simulink model "estimator_ukf"  (Simulink 7.0)
settings: Solver=FixedStepDiscrete  StartTime=1  StopTime=10.0  FixedStep=ts  RelTol=1e-3
undefined symbols (not defined in the file): c, m, magnitude, n, P0, Q, R, ROBOT, ts, W, WM, X0
libraries: simulink x5, robotics x5
settings Model: Creator=raje_ra  LastModifiedBy=raje_ra

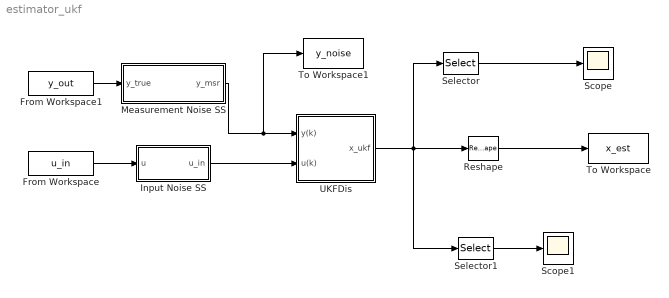
== system estimator_ukf ==
  From Workspace : FromWorkspace  VariableName=u_in  SampleTime=0
  From Workspace1 : FromWorkspace  VariableName=y_out  SampleTime=0
  Input Noise SS : Subsystem
  Measurement Noise SS : Subsystem
  Reshape : Reshape
  Scope : Scope
      settings: YMin=-2e-009  YMax=1.25e-009
  Scope1 : Scope
      settings: TimeRange=10
  Selector : Selector  InputPortWidth=62  IndexOptions=Index vector (dialog)  Indices=[1:6]  OutputSizes=1
  Selector1 : Selector  InputPortWidth=62  IndexOptions=Index vector (dialog)  Indices=[32:37]  OutputSizes=1
  To Workspace : ToWorkspace  VariableName=x_est  SampleTime=-1  SaveFormat=Structure With Time
  To Workspace1 : ToWorkspace  VariableName=y_noise  SampleTime=-1  SaveFormat=Structure With Time
  UKFDis : Subsystem
  wires:
  UKFDis/1(x_ukf) -> Selector/1, Selector1/1, Reshape/1
  From Workspace1/1 -> Measurement Noise SS/1(y_true)
  From Workspace/1 -> Input Noise SS/1(u)
  Selector/1 -> Scope/1
  Selector1/1 -> Scope1/1
  Reshape/1 -> To Workspace/1
  Measurement Noise SS/1(y_msr) -> UKFDis/1(y(k)), To Workspace1/1
  Input Noise SS/1(u_in) -> UKFDis/2(u(k))

== system estimator_ukf/Input Noise SS ==
  note: Noise with Sandard Deviation 1e-1 is added to inputs
  u : Inport  OutDataType=sfix(16)  OutScaling=2^0
  Band-Limited White Noise1 : simulink/Sources/Band-Limited White Noise  SystemSampleTime=-1  Cov=[1e-5]  Ts=ts  seed=[23341]
  Sum : Sum  Inputs=|++  OutDataType=sfix(16)  OutScaling=2^0
  u_in : Outport
  wires:
  Band-Limited White Noise1/1 -> Sum/2
  Sum/1 -> u_in/1
  u/1 -> Sum/1

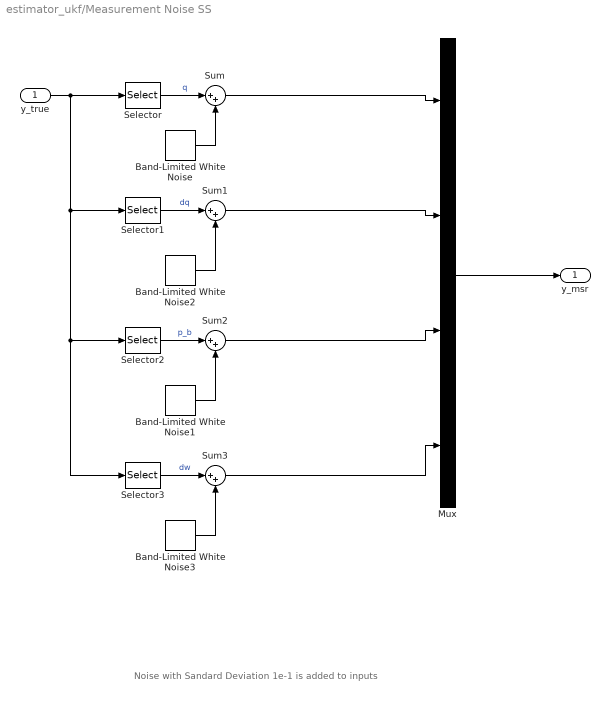
== system estimator_ukf/Measurement Noise SS ==
  note: Noise with Sandard Deviation 1e-1 is added to inputs
  y_true : Inport  OutDataType=sfix(16)  OutScaling=2^0
  Band-Limited White Noise : simulink/Sources/Band-Limited White Noise  SystemSampleTime=-1  Cov=[1e-9]  Ts=ts  seed=[23341]
  Band-Limited White Noise1 : simulink/Sources/Band-Limited White Noise  SystemSampleTime=-1  Cov=[1e-5]  Ts=ts  seed=[23341]
  Band-Limited White Noise2 : simulink/Sources/Band-Limited White Noise  SystemSampleTime=-1  Cov=[1e-7]  Ts=ts  seed=[23341]
  Band-Limited White Noise3 : simulink/Sources/Band-Limited White Noise  SystemSampleTime=-1  Cov=[1e-7]  Ts=ts  seed=[23341]
  Mux : Mux
  Selector : Selector  InputPortWidth=m  IndexOptions=Index vector (dialog)  Indices=[1:25]  OutputSizes=1
  Selector1 : Selector  InputPortWidth=m  IndexOptions=Index vector (dialog)  Indices=[26:50]  OutputSizes=1
  Selector2 : Selector  InputPortWidth=m  IndexOptions=Index vector (dialog)  Indices=[51:53]  OutputSizes=1
  Selector3 : Selector  InputPortWidth=m  IndexOptions=Index vector (dialog)  Indices=[54:56]  OutputSizes=1
  Sum{,1..3} (4 alike) : Sum  Inputs=|++  OutDataType=sfix(16)  OutScaling=2^0
  y_msr : Outport
  wires:
  Mux/1 -> y_msr/1
  Sum3/1 -> Mux/4
  Sum2/1 -> Mux/3
  Sum1/1 -> Mux/2
  Sum/1 -> Mux/1
  Selector3/1 -> Sum3/1  "dw"
  Band-Limited White Noise3/1 -> Sum3/2
  Selector2/1 -> Sum2/1  "p_b"
  Band-Limited White Noise1/1 -> Sum2/2
  Band-Limited White Noise2/1 -> Sum1/2
  Selector1/1 -> Sum1/1  "dq"
  Selector/1 -> Sum/1  "q"
  y_true/1 -> Selector3/1, Selector2/1, Selector1/1, Selector/1
  Band-Limited White Noise/1 -> Sum/2

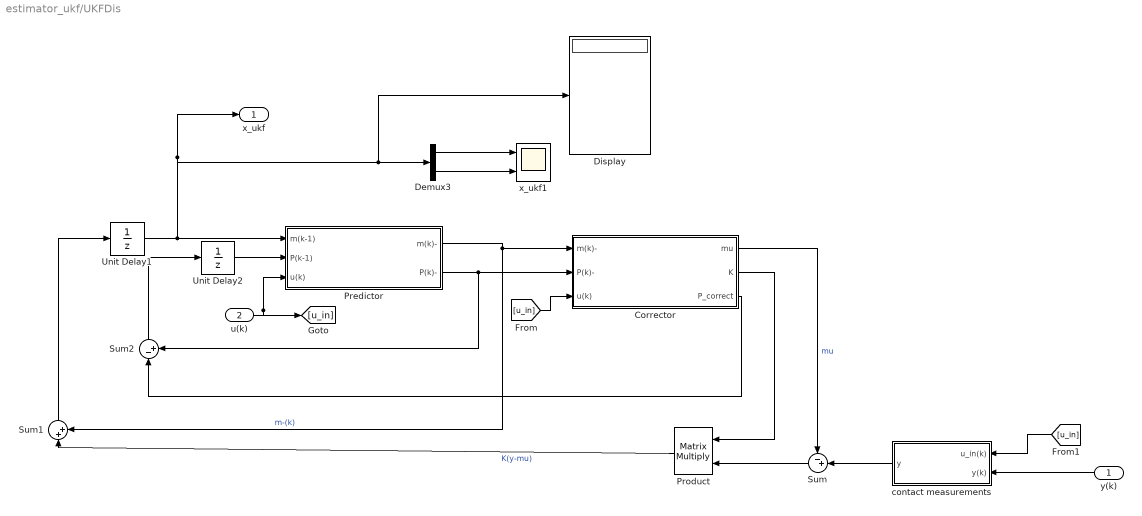
== system estimator_ukf/UKFDis ==
  y(k) : Inport  Orientation=left
  u(k) : Inport  Port=2
  Corrector : Subsystem
  Demux3 : Demux  Outputs=2
  Display : Display
  Predictor : Subsystem
  Product : Product  Orientation=left  Multiplication=Matrix(*)  OutDataType=sfix(16)  OutScaling=2^0  RndMeth=Zero
  Sum : Sum  Orientation=left  Inputs=-+|  OutDataType=sfix(16)  OutScaling=2^0
  Sum1 : Sum  Orientation=up  Inputs=|++  OutDataType=sfix(16)  OutScaling=2^0
  Sum2 : Sum  Orientation=up  Inputs=|-+  OutDataType=sfix(16)  OutScaling=2^0
  Unit Delay1 : UnitDelay  X0=X0  SampleTime=-1
  Unit Delay2 : UnitDelay  X0=P0  SampleTime=-1
  contact measurements : Subsystem  Orientation=left
  x_ukf1 : Scope  NumInputPorts=2
      settings: TimeRange=0.1  YMin=-22.5~-1.25  YMax=12.5~1.5  SaveName=ScopeData2
  x_ukf : Outport  OutDataType=sfix(16)  OutScaling=2^0
  wires:
  Demux3/1 -> x_ukf1/1
  Demux3/2 -> x_ukf1/2
  Sum1/1 -> Unit Delay1/1
  Unit Delay1/1 -> x_ukf/1, Demux3/1, Display/1, Predictor/1(m(k-1))
  Predictor/1(m(k)-) -> Sum1/2, Corrector/1(m(k)-)  "m-(k)"
  Predictor/2(P(k)-) -> Corrector/2(P(k)-), Sum2/2
  Corrector/1(mu) -> Sum/1  "mu"
  Corrector/2(K) -> Product/1
  Sum/1 -> Product/2
  Product/1 -> Sum1/1  "K(y-mu)"
  Unit Delay2/1 -> Predictor/2(P(k-1))
  Corrector/3(P_correct) -> Sum2/1
  Sum2/1 -> Unit Delay2/1
  u(k)/1 -> Predictor/3(u(k)), [u_in]
  [u_in] -> Corrector/3(u(k))
  contact measurements/1(y) -> Sum/2
  [u_in] -> contact measurements/1(u_in(k))
  y(k)/1 -> contact measurements/2(y(k))

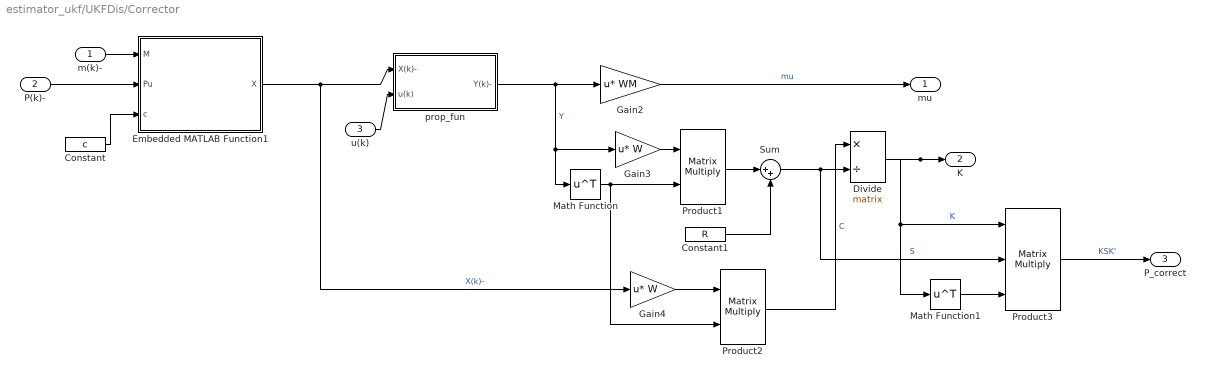
== system estimator_ukf/UKFDis/Corrector ==
  m(k)- : Inport
  P(k)- : Inport  Port=2
  u(k) : Inport  Port=3
  Constant : Constant  Value=c  OutDataType=sfix(16)  OutScaling=2^0
  Constant1 : Constant  Value=R  OutDataType=sfix(16)  OutScaling=2^0
  Divide : Product  Inputs=*/  Multiplication=Matrix(*)  OutDataType=sfix(16)  OutScaling=2^-10
  Embedded MATLAB Function1 : Stateflow chart
  Gain2 : Gain  Gain=WM  Multiplication=Matrix(u*K)  ParameterDataType=sfix(16)  ParameterScaling=2^0  OutDataType=sfix(16)  OutScaling=2^0
  Gain3 : Gain  Gain=W  Multiplication=Matrix(u*K)  ParameterDataType=sfix(16)  ParameterScaling=2^0  OutDataType=sfix(16)  OutScaling=2^0
  Gain4 : Gain  Gain=W  Multiplication=Matrix(u*K)  ParameterDataType=sfix(16)  ParameterScaling=2^0  OutDataType=sfix(16)  OutScaling=2^0
  Math Function : Math  Operator=transpose  OutDataType=sfix(16)  OutScaling=2^0  SaturateOnIntegerOverflow=on
  Math Function1 : Math  Operator=transpose  OutDataType=sfix(16)  OutScaling=2^0  SaturateOnIntegerOverflow=on
  Product1 : Product  Multiplication=Matrix(*)  OutDataType=sfix(16)  OutScaling=2^0  RndMeth=Zero
  Product2 : Product  Multiplication=Matrix(*)  OutDataType=sfix(16)  OutScaling=2^0  RndMeth=Zero
  Product3 : Product  Inputs=3  Multiplication=Matrix(*)  OutDataType=sfix(16)  OutScaling=2^0  RndMeth=Zero
  Sum : Sum  Inputs=|++  OutDataType=sfix(16)  OutScaling=2^0
  prop_fun : Subsystem
  mu : Outport
  K : Outport  Port=2
  P_correct : Outport  Port=3
  wires:
  u(k)/1 -> prop_fun/2(u(k))
  m(k)-/1 -> Embedded MATLAB Function1/1(M)
  P(k)-/1 -> Embedded MATLAB Function1/2(Pu)
  Constant/1 -> Embedded MATLAB Function1/3(c)
  Embedded MATLAB Function1/1(X) -> prop_fun/1(X(k)-), Gain4/1  "X(k)-"
  prop_fun/1(Y(k)-) -> Gain2/1, Gain3/1, Math Function/1  "Y"
  Gain2/1 -> mu/1  "mu"
  Gain3/1 -> Product1/1
  Math Function/1 -> Product1/2, Product2/2
  Product1/1 -> Sum/1
  Constant1/1 -> Sum/2
  Gain4/1 -> Product2/1
  Product2/1 -> Divide/1  "C"
  Sum/1 -> Divide/2, Product3/2  "S"
  Divide/1 -> K/1, Product3/1, Math Function1/1  "K"
  Math Function1/1 -> Product3/3
  Product3/1 -> P_correct/1  "KSK'"

== system estimator_ukf/UKFDis/Predictor ==
  m(k-1) : Inport
  P(k-1) : Inport  Port=2
  u(k) : Inport  Port=3
  Constant : Constant  Value=c  OutDataType=sfix(16)  OutScaling=2^0
  Constant1 : Constant  Value=Q  OutDataType=sfix(16)  OutScaling=2^0
  Embedded MATLAB Function1 : Stateflow chart
  Gain1 : Gain  Gain=WM  Multiplication=Matrix(u*K)  ParameterDataType=sfix(16)  ParameterScaling=2^0  OutDataType=sfix(16)  OutScaling=2^0
  Gain2 : Gain  Gain=W  Multiplication=Matrix(u*K)  ParameterDataType=sfix(16)  ParameterScaling=2^0  OutDataType=sfix(16)  OutScaling=2^0
  Math Function : Math  Operator=transpose  OutDataType=sfix(16)  OutScaling=2^0  SaturateOnIntegerOverflow=on
  Product2 : Product  Multiplication=Matrix(*)  OutDataType=sfix(16)  OutScaling=2^0  RndMeth=Zero
  Sum : Sum  Inputs=|++  OutDataType=sfix(16)  OutScaling=2^0
  prop_fun : Subsystem
  m(k)- : Outport
  P(k)- : Outport  Port=2
  wires:
  u(k)/1 -> prop_fun/2(u(k))
  Embedded MATLAB Function1/1(X) -> prop_fun/1(X(k-1))  "X(k-1)"
  Gain2/1 -> Product2/1
  Math Function/1 -> Product2/2
  Product2/1 -> Sum/1
  Constant1/1 -> Sum/2
  Sum/1 -> P(k)-/1
  Constant/1 -> Embedded MATLAB Function1/3(c)
  m(k-1)/1 -> Embedded MATLAB Function1/1(M)
  P(k-1)/1 -> Embedded MATLAB Function1/2(Pu)
  Gain1/1 -> m(k)-/1
  prop_fun/1(X(k)_hat) -> Gain2/1, Math Function/1, Gain1/1  "X(k)_hat"

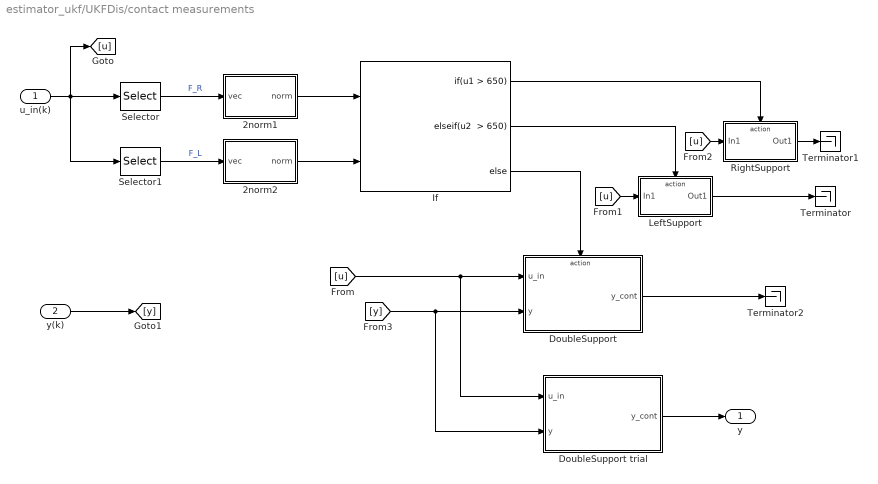
== system estimator_ukf/UKFDis/contact measurements ==
  u_in(k) : Inport
  y(k) : Inport  Port=2
  2norm1 : Subsystem
  2norm2 : Subsystem
  DoubleSupport : Subsystem  TreatAsAtomicUnit=on
  DoubleSupport trial : Subsystem  TreatAsAtomicUnit=on
  If : If  NumInputs=2  IfExpression=u1 > 650  ElseIfExpressions="u2  > 650"
  LeftSupport : Subsystem  TreatAsAtomicUnit=on
  RightSupport : Subsystem  TreatAsAtomicUnit=on
  Selector : Selector  InputPortWidth=37  IndexOptions=Index vector (dialog)  Indices=[1:3]  OutputSizes=1
  Selector1 : Selector  InputPortWidth=37  IndexOptions=Index vector (dialog)  Indices=[4:6]  OutputSizes=1
  Terminator : Terminator
  Terminator1 : Terminator
  Terminator2 : Terminator
  y : Outport
  wires:
  [y] -> DoubleSupport/2(y), DoubleSupport trial/2(y)
  y(k)/1 -> [y]
  [u] -> RightSupport/1(In1)
  [u] -> LeftSupport/1(In1)
  If/2 -> LeftSupport/Action
  If/3 -> DoubleSupport/Action
  u_in(k)/1 -> [u], Selector1/1, Selector/1
  If/1 -> RightSupport/Action
  2norm2/1(norm) -> If/2
  2norm1/1(norm) -> If/1
  Selector1/1 -> 2norm2/1(vec)  "F_L"
  Selector/1 -> 2norm1/1(vec)  "F_R"
  [u] -> DoubleSupport/1(u_in), DoubleSupport trial/1(u_in)
  RightSupport/1(Out1) -> Terminator1/1
  LeftSupport/1(Out1) -> Terminator/1
  DoubleSupport/1(y_cont) -> Terminator2/1
  DoubleSupport trial/1(y_cont) -> y/1

== system estimator_ukf/UKFDis/Corrector/prop_fun ==
  X(k)- : Inport
  u(k) : Inport  Port=2
  F(X) : Subsystem  TreatAsAtomicUnit=on
  Y(k)- : Outport
  wires:
  u(k)/1 -> F(X)/2(u(k))
  X(k)-/1 -> F(X)/1(X(k)-)
  F(X)/1(Y(k)-) -> Y(k)-/1

== system estimator_ukf/UKFDis/Predictor/prop_fun ==
  note: 1)Forward Euler Integration: x(k) = x(k-1) s*f(x(k-1))
  X(k-1) : Inport
  u(k) : Inport  Port=2
  F(X) : Subsystem  TreatAsAtomicUnit=on
  Gain3 : Gain  Gain=ts  ParameterDataType=sfix(16)  ParameterScaling=2^0  OutDataType=sfix(16)  OutScaling=2^0
  Sum1 : Sum  Inputs=|++  OutDataType=sfix(16)  OutScaling=2^0
  X(k)_hat : Outport
  wires:
  u(k)/1 -> F(X)/2(u(k))
  Sum1/1 -> X(k)_hat/1
  X(k-1)/1 -> Sum1/2, F(X)/1(X(k-1))
  F(X)/1(F(X)) -> Gain3/1
  Gain3/1 -> Sum1/1

== system estimator_ukf/UKFDis/contact measurements/2norm1 ==
  vec : Inport
  Math Function : Math  Operator=magnitude^2  OutDataType=sfix(16)  OutScaling=2^0  SaturateOnIntegerOverflow=on
  Math Function1 : Math  Operator=sqrt  OutDataType=sfix(16)  OutScaling=2^0  SaturateOnIntegerOverflow=on
  Sum of Elements : Sum  Inputs=+  OutDataType=sfix(16)  OutScaling=2^-10
  norm : Outport
  wires:
  Math Function/1 -> Sum of Elements/1
  Sum of Elements/1 -> Math Function1/1
  vec/1 -> Math Function/1
  Math Function1/1 -> norm/1

== system estimator_ukf/UKFDis/contact measurements/2norm2 ==
  vec : Inport
  Math Function : Math  Operator=magnitude^2  OutDataType=sfix(16)  OutScaling=2^0  SaturateOnIntegerOverflow=on
  Math Function1 : Math  Operator=sqrt  OutDataType=sfix(16)  OutScaling=2^0  SaturateOnIntegerOverflow=on
  Sum of Elements : Sum  Inputs=+  OutDataType=sfix(16)  OutScaling=2^-10
  norm : Outport
  wires:
  Math Function1/1 -> norm/1
  vec/1 -> Math Function/1
  Sum of Elements/1 -> Math Function1/1
  Math Function/1 -> Sum of Elements/1

== system estimator_ukf/UKFDis/contact measurements/DoubleSupport ==
  u_in : Inport  OutDataType=sfix(16)  OutScaling=2^0
  y : Inport  Port=2  OutDataType=sfix(16)  OutScaling=2^0
  Action Port : ActionPort  ActionType=else
  Constant : Constant  Value=zeros(12,1)  VectorParams1D=off  OutDataType=sfix(16)  OutScaling=2^0
  Matrix Concatenate : Concatenate  Mode=Multidimensional array
  Terminator : Terminator
  y_cont : Outport  OutDataType=sfix(16)  OutScaling=2^0
  wires:
  y/1 -> Matrix Concatenate/1
  Constant/1 -> Matrix Concatenate/2
  Matrix Concatenate/1 -> y_cont/1
  u_in/1 -> Terminator/1

== system estimator_ukf/UKFDis/contact measurements/DoubleSupport trial ==
  u_in : Inport  OutDataType=sfix(16)  OutScaling=2^0
  y : Inport  Port=2  OutDataType=sfix(16)  OutScaling=2^0
  Constant velocities : Constant  Value=zeros(12,1)  VectorParams1D=off  OutDataType=sfix(16)  OutScaling=2^0
  Constant z foot : Constant  Value=zeros(2,1)  VectorParams1D=off  OutDataType=sfix(16)  OutScaling=2^0
  Matrix Concatenate : Concatenate  NumInputs=3  Mode=Multidimensional array
  Selector : Selector  InputPortWidth=70  IndexOptions=Index vector (dialog)  Indices=[1:68]  OutputSizes=1
  Terminator : Terminator
  y_cont : Outport  OutDataType=sfix(16)  OutScaling=2^0
  wires:
  u_in/1 -> Terminator/1
  Matrix Concatenate/1 -> Selector/1
  Constant velocities/1 -> Matrix Concatenate/2
  y/1 -> Matrix Concatenate/1
  Constant z foot/1 -> Matrix Concatenate/3
  Selector/1 -> y_cont/1

== system estimator_ukf/UKFDis/contact measurements/LeftSupport ==
  In1 : Inport  OutDataType=sfix(16)  OutScaling=2^0
  Action Port : ActionPort  ActionType=elseif
  Out1 : Outport  OutDataType=sfix(16)  OutScaling=2^0
  wires:
  In1/1 -> Out1/1

== system estimator_ukf/UKFDis/contact measurements/RightSupport ==
  In1 : Inport  OutDataType=sfix(16)  OutScaling=2^0
  Action Port : ActionPort  ActionType=then
  Out1 : Outport  OutDataType=sfix(16)  OutScaling=2^0
  wires:
  In1/1 -> Out1/1

== system estimator_ukf/UKFDis/Corrector/prop_fun/F(X) ==
  X(k)- : Inport  OutDataType=sfix(16)  OutScaling=2^0
  u(k) : Inport  Port=2  OutDataType=sfix(16)  OutScaling=2^0
  Assignment : Assignment  NumberOfDimensions=2  IndexOptions=Assign all,Index vector (port)  Indices=1,1  OutputSizes=2,2
  Constant : Constant  Value=zeros(m+12,2*n+1)  VectorParams1D=off  OutDataType=sfix(16)  OutScaling=2^0  SampleTime=-1
  Display : Display
  For Iterator : ForIterator  ResetStates=reset  IterationLimit=2*n +1  IterationVariableDataType=double
  Measurements : Subsystem
  Selector : Selector  NumberOfDimensions=2  IndexOptions=Select all,Index vector (port)  Indices=[1 3],1  OutputSizes=1,1
  Y(k)- : Outport  OutDataType=sfix(16)  OutScaling=2^0
  wires:
  u(k)/1 -> Measurements/2(u)
  Constant/1 -> Assignment/1
  Assignment/1 -> Y(k)-/1
  Measurements/1(y) -> Assignment/2
  Selector/1 -> Measurements/1(x)
  For Iterator/1 -> Display/1, Assignment/3, Selector/2
  X(k)-/1 -> Selector/1

== system estimator_ukf/UKFDis/Predictor/prop_fun/F(X) ==
  X(k-1) : Inport  OutDataType=sfix(16)  OutScaling=2^0
  u(k) : Inport  Port=2  OutDataType=sfix(16)  OutScaling=2^0
  Assignment : Assignment  NumberOfDimensions=2  IndexOptions=Assign all,Index vector (port)  Indices=1,1  OutputSizes=2,2
  For Iterator : ForIterator  ResetStates=reset  IterationLimit=2*n +1  IterationVariableDataType=double
  Selector : Selector  NumberOfDimensions=2  IndexOptions=Select all,Index vector (port)  Indices=[1 3],1  OutputSizes=1,1
  dyn_model : Subsystem
  F(X) : Outport  OutDataType=sfix(16)  OutScaling=2^0
  wires:
  Assignment/1 -> F(X)/1
  dyn_model/1(f(x(k-1))) -> Assignment/2
  Selector/1 -> dyn_model/1(x(k-1))
  For Iterator/1 -> Selector/2, Assignment/3
  X(k-1)/1 -> Assignment/1, Selector/1
  u(k)/1 -> dyn_model/2(u_in(k))

== system estimator_ukf/UKFDis/Corrector/prop_fun/F(X)/Measurements ==
  x : Inport
  u : Inport  Port=2
  Matrix Concatenate : Concatenate  NumInputs=5  Mode=Multidimensional array
  dq : Selector  InputPortWidth=62  IndexOptions=Index vector (dialog)  Indices=[38:62]  OutputSizes=1
  dyn_model : Subsystem
  q : Selector  InputPortWidth=62  IndexOptions=Index vector (dialog)  Indices=[7:31]  OutputSizes=1
  y : Outport  OutDataType=sfix(16)  OutScaling=2^0
  wires:
  Matrix Concatenate/1 -> y/1
  x/1 -> q/1, dq/1, dyn_model/1(x(k-1))
  u/1 -> dyn_model/2(u_in(k))
  dyn_model/1(acc(k)) -> Matrix Concatenate/3
  q/1 -> Matrix Concatenate/1
  dq/1 -> Matrix Concatenate/2
  dyn_model/3(v_cont) -> Matrix Concatenate/5
  dyn_model/2(gyro) -> Matrix Concatenate/4

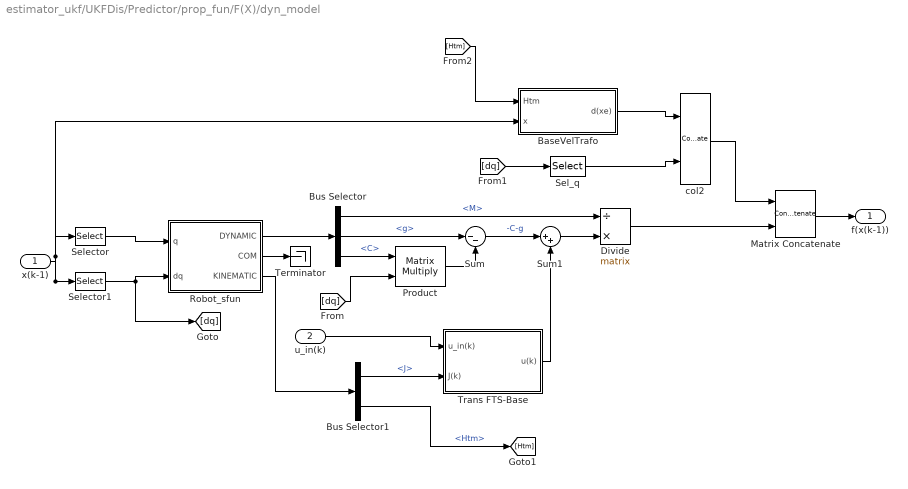
== system estimator_ukf/UKFDis/Predictor/prop_fun/F(X)/dyn_model ==
  x(k-1) : Inport
  u_in(k) : Inport  Port=2
  BaseVelTrafo : Subsystem
  Bus Selector : BusSelector  OutputSignals=M,g,C
  Bus Selector1 : BusSelector  OutputSignals=J,Htm
  Divide : Product  Inputs=/*  Multiplication=Matrix(*)  OutDataType=sfix(16)  OutScaling=2^-10
  Matrix Concatenate : Concatenate  Mode=Multidimensional array
  Product : Product  Multiplication=Matrix(*)  OutDataType=sfix(16)  OutScaling=2^0  RndMeth=Zero
  Robot_sfun : Subsystem
  Sel_q : Selector  InputPortWidth=31  IndexOptions=Index vector (dialog)  Indices=[7:31]  OutputSizes=1
  Selector : Selector  InputPortWidth=62  IndexOptions=Index vector (dialog)  Indices=[1:31]  OutputSizes=1
  Selector1 : Selector  InputPortWidth=62  IndexOptions=Index vector (dialog)  Indices=[32:62]  OutputSizes=1
  Sum : Sum  Inputs=|--  OutDataType=sfix(16)  OutScaling=2^0
  Sum1 : Sum  Inputs=|++  OutDataType=sfix(16)  OutScaling=2^0
  Terminator : Terminator
  Trans FTS-Base : Subsystem
  col2 : Concatenate  Mode=Multidimensional array
  f(x(k-1)) : Outport
  wires:
  Robot_sfun/1(DYNAMIC) -> Bus Selector/1
  Bus Selector/3 -> Product/1  "<C>"
  [dq] -> Product/2
  Product/1 -> Sum/2
  Bus Selector/2 -> Sum/1  "<g>"
  Sum/1 -> Sum1/1  "-C-g"
  Bus Selector/1 -> Divide/1  "<M>"
  Sum1/1 -> Divide/2
  Robot_sfun/3(KINEMATIC) -> Bus Selector1/1
  x(k-1)/1 -> Selector/1, Selector1/1, BaseVelTrafo/2(x)
  Selector/1 -> Robot_sfun/1(q)
  Selector1/1 -> Robot_sfun/2(dq), [dq]
  Robot_sfun/2(COM) -> Terminator/1
  Matrix Concatenate/1 -> f(x(k-1))/1
  Divide/1 -> Matrix Concatenate/2
  Bus Selector1/1 -> Trans FTS-Base/2(J(k))  "<J>"
  u_in(k)/1 -> Trans FTS-Base/1(u_in(k))
  Trans FTS-Base/1(u(k)) -> Sum1/2
  Bus Selector1/2 -> [Htm]  "<Htm>"
  [Htm] -> BaseVelTrafo/1(Htm)
  BaseVelTrafo/1(d(xe)) -> col2/1
  [dq] -> Sel_q/1
  Sel_q/1 -> col2/2
  col2/1 -> Matrix Concatenate/1

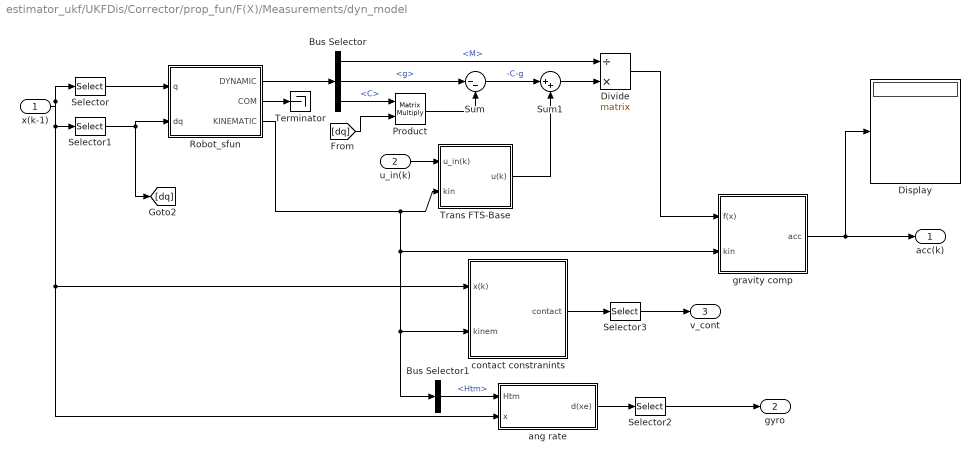
== system estimator_ukf/UKFDis/Corrector/prop_fun/F(X)/Measurements/dyn_model ==
  x(k-1) : Inport
  u_in(k) : Inport  Port=2
  Bus Selector : BusSelector  OutputSignals=M,g,C
  Bus Selector1 : BusSelector  OutputSignals=Htm
  Display : Display
  Divide : Product  Inputs=/*  Multiplication=Matrix(*)  OutDataType=sfix(16)  OutScaling=2^-10
  Product : Product  Multiplication=Matrix(*)  OutDataType=sfix(16)  OutScaling=2^0  RndMeth=Zero
  Robot_sfun : Subsystem
  Selector : Selector  InputPortWidth=62  IndexOptions=Index vector (dialog)  Indices=[1:31]  OutputSizes=1
  Selector1 : Selector  InputPortWidth=62  IndexOptions=Index vector (dialog)  Indices=[32:62]  OutputSizes=1
  Selector2 : Selector  InputPortWidth=6  IndexOptions=Index vector (dialog)  Indices=[4:6]  OutputSizes=1
  Selector3 : Selector  InputPortWidth=14  IndexOptions=Index vector (dialog)  Indices=[1:12]  OutputSizes=1
  Sum : Sum  Inputs=|--  OutDataType=sfix(16)  OutScaling=2^0
  Sum1 : Sum  Inputs=|++  OutDataType=sfix(16)  OutScaling=2^0
  Terminator : Terminator
  Trans FTS-Base : Subsystem
  ang rate : Subsystem
  contact constranints : Subsystem
  gravity comp : Subsystem
  acc(k) : Outport
  gyro : Outport  Port=2
  v_cont : Outport  Port=3
  wires:
  Robot_sfun/1(DYNAMIC) -> Bus Selector/1
  Bus Selector/3 -> Product/1  "<C>"
  [dq] -> Product/2
  Product/1 -> Sum/2
  Bus Selector/2 -> Sum/1  "<g>"
  Sum/1 -> Sum1/1  "-C-g"
  Bus Selector/1 -> Divide/1  "<M>"
  Sum1/1 -> Divide/2
  Robot_sfun/3(KINEMATIC) -> Trans FTS-Base/2(kin), gravity comp/2(kin), contact constranints/2(kinem), Bus Selector1/1
  x(k-1)/1 -> Selector/1, Selector1/1, contact constranints/1(x(k)), ang rate/2(x)
  Selector/1 -> Robot_sfun/1(q)
  Selector1/1 -> Robot_sfun/2(dq), [dq]
  Robot_sfun/2(COM) -> Terminator/1
  u_in(k)/1 -> Trans FTS-Base/1(u_in(k))
  Trans FTS-Base/1(u(k)) -> Sum1/2
  Divide/1 -> gravity comp/1(f(x))
  gravity comp/1(acc) -> acc(k)/1, Display/1
  contact constranints/1(contact) -> Selector3/1
  Bus Selector1/1 -> ang rate/1(Htm)  "<Htm>"
  ang rate/1(d(xe)) -> Selector2/1
  Selector2/1 -> gyro/1
  Selector3/1 -> v_cont/1

== system estimator_ukf/UKFDis/Predictor/prop_fun/F(X)/dyn_model/BaseVelTrafo ==
  note: xe = [pos of endeffector, ori of endeffector]
  Htm : Inport
  x : Inport  Port=2
  Divide : Product  Inputs=/**  Multiplication=Matrix(*)  OutDataType=sfix(16)  OutScaling=2^-10
  H_sb : Selector  NumberOfDimensions=2  InputPortWidth=31  IndexOptions=Index vector (dialog),Select all  Indices=[17:20],[1:3]  OutputSizes=1,1
  Selector : Selector  InputPortWidth=62  IndexOptions=Index vector (dialog)  Indices=[32:37]  OutputSizes=1
  Selector5 : Selector  InputPortWidth=62  IndexOptions=Index vector (dialog)  Indices=[4:6]  OutputSizes=1
  T : Subsystem
  Tdisp : Display
  Trafo3D Adjoint : robotics/Trafo3D Adjoint  SystemSampleTime=-1
  d(xe) disp : Display
  velbase disp : Display
  d(xe) : Outport
  wires:
  Selector/1 -> Divide/3, velbase disp/1  "v_b"
  T/1(T) -> Tdisp/1, Divide/1
  H_sb/1 -> Trafo3D Adjoint/1
  x/1 -> Selector/1, Selector5/1
  Divide/1 -> d(xe) disp/1, d(xe)/1
  Selector5/1 -> T/1(eulVec)
  Htm/1 -> H_sb/1
  Trafo3D Adjoint/1 -> Divide/2

== system estimator_ukf/UKFDis/Predictor/prop_fun/F(X)/dyn_model/Robot_sfun ==
  q : Inport
  dq : Inport  Port=2
  Bus Creator : BusCreator
  Bus Creator1 : BusCreator  Inputs=3
  Bus Creator2 : BusCreator  Inputs=3
  S-Function : S-Function  FunctionName=luca_dynamics_sfun  Parameters=(size(ROBOT.csi,1)/6-1), size(ROBOT.csi,2), ROBOT.parent, ROBOT.tcp, ROBOT.g0, ROBOT.csi, ROBOT.com, ROBOT.Mass
  DYNAMIC : Outport
  COM : Outport  Port=2
  KINEMATIC : Outport  Port=3
  wires:
  q/1 -> S-Function/1
  dq/1 -> S-Function/2
  S-Function/1 -> Bus Creator/1  "M"
  S-Function/2 -> Bus Creator/2  "C"
  S-Function/3 -> Bus Creator/3  "g"
  S-Function/4 -> Bus Creator/4  "dM"
  S-Function/5 -> Bus Creator1/1  "x"
  S-Function/6 -> Bus Creator1/2  "J"
  S-Function/7 -> Bus Creator1/3  "dJ"
  S-Function/8 -> Bus Creator2/1  "Htm"
  S-Function/9 -> Bus Creator2/2  "J"
  S-Function/10 -> Bus Creator2/3  "dJ"
  Bus Creator/1 -> DYNAMIC/1
  Bus Creator1/1 -> COM/1
  Bus Creator2/1 -> KINEMATIC/1

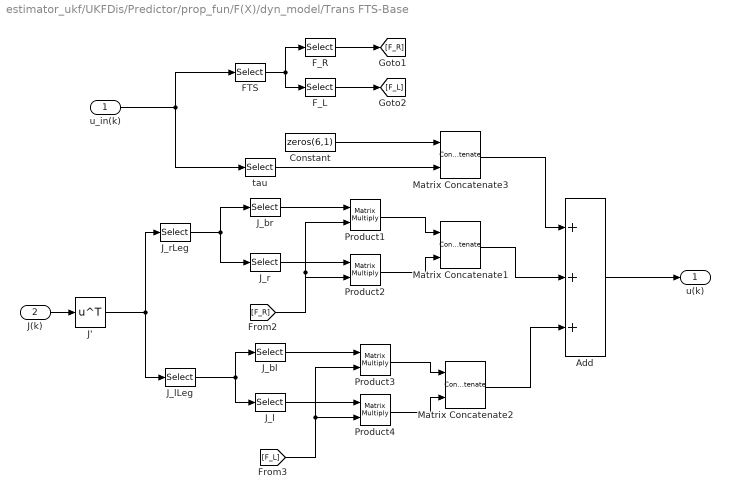
== system estimator_ukf/UKFDis/Predictor/prop_fun/F(X)/dyn_model/Trans FTS-Base ==
  u_in(k) : Inport
  J(k) : Inport  Port=2
  Add : Sum  Inputs=+++  OutDataType=sfix(16)  OutScaling=2^-10
  Constant : Constant  Value=zeros(6,1)  VectorParams1D=off  OutDataType=sfix(16)  OutScaling=2^0
  FTS : Selector  InputPortWidth=37  IndexOptions=Index vector (dialog)  Indices=[1:12]  OutputSizes=1
  F_L : Selector  InputPortWidth=12  IndexOptions=Index vector (dialog)  Indices=[7:12]  OutputSizes=1
  F_R : Selector  InputPortWidth=12  IndexOptions=Index vector (dialog)  Indices=[1:6]  OutputSizes=1
  J' : Math  Operator=transpose  OutDataType=sfix(16)  OutScaling=2^0  SaturateOnIntegerOverflow=on
  J_bl : Selector  NumberOfDimensions=2  InputPortWidth=37  IndexOptions=Index vector (dialog),Select all  Indices=[1:6],  OutputSizes=1,1
  J_br : Selector  NumberOfDimensions=2  InputPortWidth=37  IndexOptions=Index vector (dialog),Select all  Indices=[1:6],  OutputSizes=1,1
  J_l : Selector  NumberOfDimensions=2  InputPortWidth=37  IndexOptions=Index vector (dialog),Select all  Indices=[7:31],  OutputSizes=1,1
  J_lLeg : Selector  NumberOfDimensions=2  InputPortWidth=37  IndexOptions=Select all,Index vector (dialog)  Indices=[7:12],[7:12]  OutputSizes=1,1
  J_r : Selector  NumberOfDimensions=2  InputPortWidth=37  IndexOptions=Index vector (dialog),Select all  Indices=[7:31],  OutputSizes=1,1
  J_rLeg : Selector  NumberOfDimensions=2  InputPortWidth=37  IndexOptions=Select all,Index vector (dialog)  Indices=,[1:6]  OutputSizes=1,1
  Matrix Concatenate1 : Concatenate  Mode=Multidimensional array
  Matrix Concatenate2 : Concatenate  Mode=Multidimensional array
  Matrix Concatenate3 : Concatenate  Mode=Multidimensional array
  Product{1..4} (4 alike) : Product  Multiplication=Matrix(*)  OutDataType=sfix(16)  OutScaling=2^0  RndMeth=Zero
  tau : Selector  InputPortWidth=37  IndexOptions=Index vector (dialog)  Indices=[13:37]  OutputSizes=1
  u(k) : Outport
  wires:
  u_in(k)/1 -> FTS/1, tau/1
  J_rLeg/1 -> J_br/1, J_r/1
  J_lLeg/1 -> J_bl/1, J_l/1
  FTS/1 -> F_R/1, F_L/1
  F_R/1 -> [F_R]
  F_L/1 -> [F_L]
  J'/1 -> J_rLeg/1, J_lLeg/1
  J_br/1 -> Product1/1
  [F_R] -> Product1/2, Product2/2
  J_r/1 -> Product2/1
  J_bl/1 -> Product3/1
  [F_L] -> Product3/2, Product4/2
  J_l/1 -> Product4/1
  Product3/1 -> Matrix Concatenate2/1
  Product4/1 -> Matrix Concatenate2/2
  Product1/1 -> Matrix Concatenate1/1
  Product2/1 -> Matrix Concatenate1/2
  J(k)/1 -> J'/1
  tau/1 -> Matrix Concatenate3/2
  Constant/1 -> Matrix Concatenate3/1
  Matrix Concatenate3/1 -> Add/1
  Matrix Concatenate1/1 -> Add/2
  Matrix Concatenate2/1 -> Add/3
  Add/1 -> u(k)/1

== system estimator_ukf/UKFDis/Corrector/prop_fun/F(X)/Measurements/dyn_model/Robot_sfun ==
  q : Inport
  dq : Inport  Port=2
  Bus Creator : BusCreator
  Bus Creator1 : BusCreator  Inputs=3
  Bus Creator2 : BusCreator  Inputs=3
  S-Function : S-Function  FunctionName=luca_dynamics_sfun  Parameters=(size(ROBOT.csi,1)/6-1), size(ROBOT.csi,2), ROBOT.parent, ROBOT.tcp, ROBOT.g0, ROBOT.csi, ROBOT.com, ROBOT.Mass
  DYNAMIC : Outport
  COM : Outport  Port=2
  KINEMATIC : Outport  Port=3
  wires:
  q/1 -> S-Function/1
  dq/1 -> S-Function/2
  S-Function/1 -> Bus Creator/1  "M"
  S-Function/2 -> Bus Creator/2  "C"
  S-Function/3 -> Bus Creator/3  "g"
  S-Function/4 -> Bus Creator/4  "dM"
  S-Function/5 -> Bus Creator1/1  "x"
  S-Function/6 -> Bus Creator1/2  "J"
  S-Function/7 -> Bus Creator1/3  "dJ"
  S-Function/8 -> Bus Creator2/1  "Htm"
  S-Function/9 -> Bus Creator2/2  "J"
  S-Function/10 -> Bus Creator2/3  "dJ"
  Bus Creator/1 -> DYNAMIC/1
  Bus Creator1/1 -> COM/1
  Bus Creator2/1 -> KINEMATIC/1

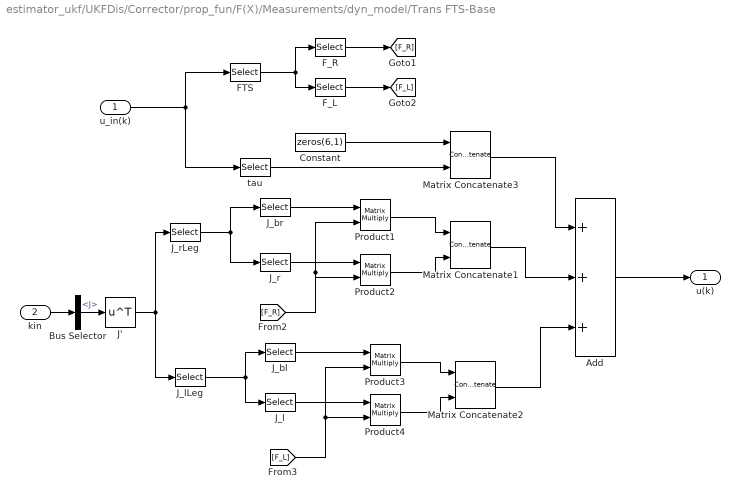
== system estimator_ukf/UKFDis/Corrector/prop_fun/F(X)/Measurements/dyn_model/Trans FTS-Base ==
  u_in(k) : Inport
  kin : Inport  Port=2
  Add : Sum  Inputs=+++  OutDataType=sfix(16)  OutScaling=2^-10
  Bus Selector : BusSelector  OutputSignals=J
  Constant : Constant  Value=zeros(6,1)  VectorParams1D=off  OutDataType=sfix(16)  OutScaling=2^0
  FTS : Selector  InputPortWidth=37  IndexOptions=Index vector (dialog)  Indices=[1:12]  OutputSizes=1
  F_L : Selector  InputPortWidth=12  IndexOptions=Index vector (dialog)  Indices=[7:12]  OutputSizes=1
  F_R : Selector  InputPortWidth=12  IndexOptions=Index vector (dialog)  Indices=[1:6]  OutputSizes=1
  J' : Math  Operator=transpose  OutDataType=sfix(16)  OutScaling=2^0  SaturateOnIntegerOverflow=on
  J_bl : Selector  NumberOfDimensions=2  InputPortWidth=37  IndexOptions=Index vector (dialog),Select all  Indices=[1:6],  OutputSizes=1,1
  J_br : Selector  NumberOfDimensions=2  InputPortWidth=37  IndexOptions=Index vector (dialog),Select all  Indices=[1:6],  OutputSizes=1,1
  J_l : Selector  NumberOfDimensions=2  InputPortWidth=37  IndexOptions=Index vector (dialog),Select all  Indices=[7:31],  OutputSizes=1,1
  J_lLeg : Selector  NumberOfDimensions=2  InputPortWidth=37  IndexOptions=Select all,Index vector (dialog)  Indices=[7:12],[7:12]  OutputSizes=1,1
  J_r : Selector  NumberOfDimensions=2  InputPortWidth=37  IndexOptions=Index vector (dialog),Select all  Indices=[7:31],  OutputSizes=1,1
  J_rLeg : Selector  NumberOfDimensions=2  InputPortWidth=37  IndexOptions=Select all,Index vector (dialog)  Indices=,[1:6]  OutputSizes=1,1
  Matrix Concatenate1 : Concatenate  Mode=Multidimensional array
  Matrix Concatenate2 : Concatenate  Mode=Multidimensional array
  Matrix Concatenate3 : Concatenate  Mode=Multidimensional array
  Product{1..4} (4 alike) : Product  Multiplication=Matrix(*)  OutDataType=sfix(16)  OutScaling=2^0  RndMeth=Zero
  tau : Selector  InputPortWidth=37  IndexOptions=Index vector (dialog)  Indices=[13:37]  OutputSizes=1
  u(k) : Outport
  wires:
  u_in(k)/1 -> FTS/1, tau/1
  J_rLeg/1 -> J_br/1, J_r/1
  J_lLeg/1 -> J_bl/1, J_l/1
  FTS/1 -> F_R/1, F_L/1
  F_R/1 -> [F_R]
  F_L/1 -> [F_L]
  J'/1 -> J_rLeg/1, J_lLeg/1
  J_br/1 -> Product1/1
  [F_R] -> Product1/2, Product2/2
  J_r/1 -> Product2/1
  J_bl/1 -> Product3/1
  [F_L] -> Product3/2, Product4/2
  J_l/1 -> Product4/1
  Product3/1 -> Matrix Concatenate2/1
  Product4/1 -> Matrix Concatenate2/2
  Product1/1 -> Matrix Concatenate1/1
  Product2/1 -> Matrix Concatenate1/2
  tau/1 -> Matrix Concatenate3/2
  Constant/1 -> Matrix Concatenate3/1
  Matrix Concatenate3/1 -> Add/1
  Matrix Concatenate1/1 -> Add/2
  Matrix Concatenate2/1 -> Add/3
  Add/1 -> u(k)/1
  kin/1 -> Bus Selector/1
  Bus Selector/1 -> J'/1  "<J>"

== system estimator_ukf/UKFDis/Corrector/prop_fun/F(X)/Measurements/dyn_model/ang rate ==
  note: xe = [pos of endeffector, ori of endeffector]
  Htm : Inport
  x : Inport  Port=2
  Divide : Product  Inputs=/**  Multiplication=Matrix(*)  OutDataType=sfix(16)  OutScaling=2^-10
  H_sb : Selector  NumberOfDimensions=2  InputPortWidth=31  IndexOptions=Index vector (dialog),Select all  Indices=[17:20],[1:3]  OutputSizes=1,1
  Product : Product  Multiplication=Matrix(*)  OutDataType=sfix(16)  OutScaling=2^0  RndMeth=Zero
  Selector : Selector  InputPortWidth=62  IndexOptions=Index vector (dialog)  Indices=[32:37]  OutputSizes=1
  Selector5 : Selector  InputPortWidth=62  IndexOptions=Index vector (dialog)  Indices=[4:6]  OutputSizes=1
  T : Subsystem
  Tdisp : Display
  Trafo3D Adjoint : robotics/Trafo3D Adjoint  SystemSampleTime=-1
  Trafo3D Inverse Adjoint : Subsystem
      mask Description: Adjoint matrix for a given frame.
  d(xe) disp : Display
  velbase disp : Display
  d(xe) : Outport
  wires:
  Selector/1 -> Divide/3, velbase disp/1  "v_b"
  T/1(T) -> Tdisp/1, Divide/1
  H_sb/1 -> Trafo3D Adjoint/1, Trafo3D Inverse Adjoint/1(H)
  x/1 -> Selector/1, Selector5/1
  Divide/1 -> Product/2
  Selector5/1 -> T/1(eulVec)
  Htm/1 -> H_sb/1
  Trafo3D Adjoint/1 -> Divide/2
  Trafo3D Inverse Adjoint/1(inv(AdH)) -> Product/1
  Product/1 -> d(xe)/1, d(xe) disp/1

== system estimator_ukf/UKFDis/Corrector/prop_fun/F(X)/Measurements/dyn_model/contact constranints ==
  x(k) : Inport
  kinem : Inport  Port=2
  Display : Display
  Display1 : Display
  DoubleSupport : Subsystem  TreatAsAtomicUnit=on
  Matrix Concatenate : Concatenate  NumInputs=3  Mode=Multidimensional array
  contact : Outport
  wires:
  kinem/1 -> DoubleSupport/2(kinematics)
  x(k)/1 -> DoubleSupport/1(x(k))
  DoubleSupport/1(V_r) -> Matrix Concatenate/1, Display1/1
  DoubleSupport/2(V_l) -> Matrix Concatenate/2
  Matrix Concatenate/1 -> contact/1
  DoubleSupport/3(p_z) -> Display/1, Matrix Concatenate/3

== system estimator_ukf/UKFDis/Corrector/prop_fun/F(X)/Measurements/dyn_model/gravity comp ==
  note: Acc _spacial = Ad_g * Acc_body
  f(x) : Inport
  kin : Inport  Port=2
  Bus Selector : BusSelector  OutputSignals=Htm
  Display : Display
  H2Rp : robotics/H2Rp  SystemSampleTime=-1
  Math Function : Math  Operator=transpose  OutDataType=sfix(16)  OutScaling=2^0  SaturateOnIntegerOverflow=on
  Product : Product  Multiplication=Matrix(*)  OutDataType=sfix(16)  OutScaling=2^0  RndMeth=Zero
  Sum : Sum  Inputs=|++  OutDataType=sfix(16)  OutScaling=2^0
  Terminator : Terminator
  acc1 : Constant  Value=[0 0 9.81]'  VectorParams1D=off  OutDataType=sfix(16)  OutScaling=2^0
  ddx : Selector  InputPortWidth=31  IndexOptions=Index vector (dialog)  Indices=[1:3]  OutputSizes=1
  ddx2 : Selector  NumberOfDimensions=2  InputPortWidth=31  IndexOptions=Index vector (dialog),Select all  Indices=[17:20],1  OutputSizes=1,1
  acc : Outport
  wires:
  f(x)/1 -> ddx/1
  kin/1 -> Bus Selector/1
  Bus Selector/1 -> ddx2/1  "<Htm>"
  ddx2/1 -> H2Rp/1, Display/1
  Product/1 -> Sum/1
  ddx/1 -> Sum/2  "acc"
  Sum/1 -> acc/1
  H2Rp/1 -> Math Function/1
  H2Rp/2 -> Terminator/1
  Math Function/1 -> Product/1
  acc1/1 -> Product/2  "gravity"

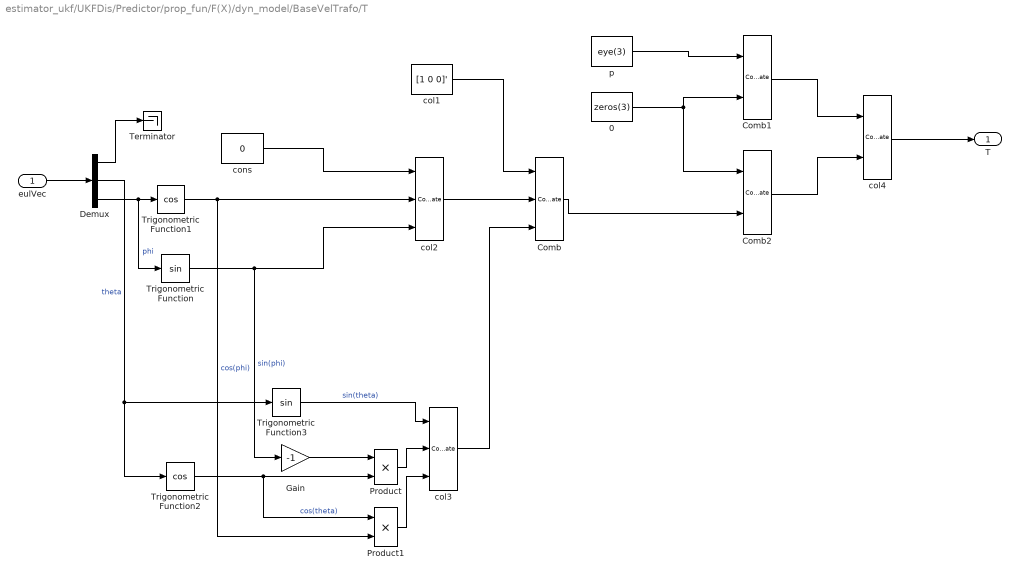
== system estimator_ukf/UKFDis/Predictor/prop_fun/F(X)/dyn_model/BaseVelTrafo/T ==
  eulVec : Inport
  0 : Constant  Value=zeros(3)  VectorParams1D=off  OutDataType=sfix(16)  OutScaling=2^0
  Comb : Concatenate  NumInputs=3  Mode=Multidimensional array  ConcatenateDimension=2
  Comb1 : Concatenate  Mode=Multidimensional array  ConcatenateDimension=2
  Comb2 : Concatenate  Mode=Multidimensional array  ConcatenateDimension=2
  Demux : Demux  Outputs=3
  Gain : Gain  Gain=-1  ParameterDataType=sfix(16)  ParameterScaling=2^0  OutDataType=sfix(16)  OutScaling=2^0
  Product : Product  OutDataType=sfix(16)  OutScaling=2^0  RndMeth=Zero
  Product1 : Product  OutDataType=sfix(16)  OutScaling=2^0  RndMeth=Zero
  Terminator : Terminator
  Trigonometric Function : Trigonometry
  Trigonometric Function1 : Trigonometry  Operator=cos
  Trigonometric Function2 : Trigonometry  Operator=cos
  Trigonometric Function3 : Trigonometry
  col1 : Constant  Value=[1 0 0]'  VectorParams1D=off  OutDataType=sfix(16)  OutScaling=2^0
  col2 : Concatenate  NumInputs=3  Mode=Multidimensional array
  col3 : Concatenate  NumInputs=3  Mode=Multidimensional array
  col4 : Concatenate  Mode=Multidimensional array
  cons : Constant  Value=0  VectorParams1D=off  OutDataType=sfix(16)  OutScaling=2^0
  p : Constant  Value=eye(3)  VectorParams1D=off  OutDataType=sfix(16)  OutScaling=2^0
  T : Outport
  wires:
  col3/1 -> Comb/3
  Product1/1 -> col3/3
  Product/1 -> col3/2
  Gain/1 -> Product/1
  Trigonometric Function3/1 -> col3/1  "sin(theta)"
  Demux/1 -> Terminator/1
  col2/1 -> Comb/2
  col1/1 -> Comb/1
  Trigonometric Function2/1 -> Product1/1, Product/2  "cos(theta)"
  Demux/2 -> Trigonometric Function3/1, Trigonometric Function2/1  "theta"
  cons/1 -> col2/1
  Trigonometric Function/1 -> Gain/1, col2/3  "sin(phi)"
  Trigonometric Function1/1 -> col2/2, Product1/2  "cos(phi)"
  Demux/3 -> Trigonometric Function/1, Trigonometric Function1/1  "phi"
  eulVec/1 -> Demux/1
  p/1 -> Comb1/1
  0/1 -> Comb1/2, Comb2/1
  Comb/1 -> Comb2/2
  Comb1/1 -> col4/1
  Comb2/1 -> col4/2
  col4/1 -> T/1

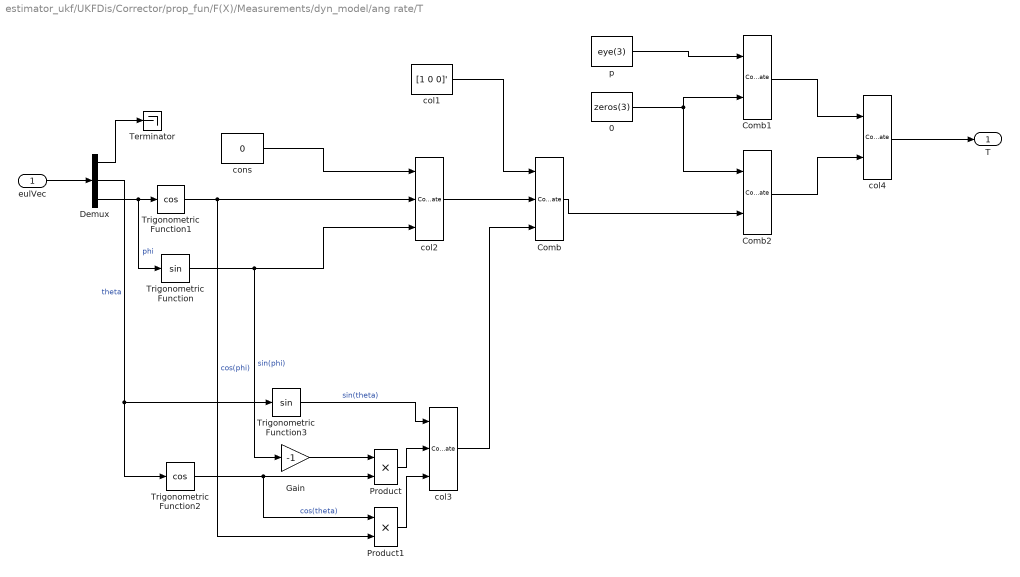
== system estimator_ukf/UKFDis/Corrector/prop_fun/F(X)/Measurements/dyn_model/ang rate/T ==
  eulVec : Inport
  0 : Constant  Value=zeros(3)  VectorParams1D=off  OutDataType=sfix(16)  OutScaling=2^0
  Comb : Concatenate  NumInputs=3  Mode=Multidimensional array  ConcatenateDimension=2
  Comb1 : Concatenate  Mode=Multidimensional array  ConcatenateDimension=2
  Comb2 : Concatenate  Mode=Multidimensional array  ConcatenateDimension=2
  Demux : Demux  Outputs=3
  Gain : Gain  Gain=-1  ParameterDataType=sfix(16)  ParameterScaling=2^0  OutDataType=sfix(16)  OutScaling=2^0
  Product : Product  OutDataType=sfix(16)  OutScaling=2^0  RndMeth=Zero
  Product1 : Product  OutDataType=sfix(16)  OutScaling=2^0  RndMeth=Zero
  Terminator : Terminator
  Trigonometric Function : Trigonometry
  Trigonometric Function1 : Trigonometry  Operator=cos
  Trigonometric Function2 : Trigonometry  Operator=cos
  Trigonometric Function3 : Trigonometry
  col1 : Constant  Value=[1 0 0]'  VectorParams1D=off  OutDataType=sfix(16)  OutScaling=2^0
  col2 : Concatenate  NumInputs=3  Mode=Multidimensional array
  col3 : Concatenate  NumInputs=3  Mode=Multidimensional array
  col4 : Concatenate  Mode=Multidimensional array
  cons : Constant  Value=0  VectorParams1D=off  OutDataType=sfix(16)  OutScaling=2^0
  p : Constant  Value=eye(3)  VectorParams1D=off  OutDataType=sfix(16)  OutScaling=2^0
  T : Outport
  wires:
  col3/1 -> Comb/3
  Product1/1 -> col3/3
  Product/1 -> col3/2
  Gain/1 -> Product/1
  Trigonometric Function3/1 -> col3/1  "sin(theta)"
  Demux/1 -> Terminator/1
  col2/1 -> Comb/2
  col1/1 -> Comb/1
  Trigonometric Function2/1 -> Product1/1, Product/2  "cos(theta)"
  Demux/2 -> Trigonometric Function3/1, Trigonometric Function2/1  "theta"
  cons/1 -> col2/1
  Trigonometric Function/1 -> Gain/1, col2/3  "sin(phi)"
  Trigonometric Function1/1 -> col2/2, Product1/2  "cos(phi)"
  Demux/3 -> Trigonometric Function/1, Trigonometric Function1/1  "phi"
  eulVec/1 -> Demux/1
  p/1 -> Comb1/1
  0/1 -> Comb1/2, Comb2/1
  Comb/1 -> Comb2/2
  Comb1/1 -> col4/1
  Comb2/1 -> col4/2
  col4/1 -> T/1

== system estimator_ukf/UKFDis/Corrector/prop_fun/F(X)/Measurements/dyn_model/ang rate/Trafo3D Inverse Adjoint ==
  H : Inport  OutDataType=sfix(16)  OutScaling=2^0
  0 : Constant  Value=zeros(3,3)  VectorParams1D=off  OutDataType=sfix(16)  OutScaling=2^0
  Cross-Product : Subsystem  AncestorBlock=robotics/Cross-Product
      mask Description: Vector Cross Product, compatible also with matrices: out = crossProduct(v, m), where m may be a vector or a 3xn matrix
  Gain : Gain  Gain=-1  ParameterDataType=sfix(16)  ParameterScaling=2^0  OutDataType=sfix(16)  OutScaling=2^0
  Math Function : Math  Operator=transpose  OutDataType=sfix(16)  OutScaling=2^0  SaturateOnIntegerOverflow=on
  Matrix Concatenation : Concatenate  Mode=Multidimensional array  ConcatenateDimension=2
  Matrix Concatenation1 : Concatenate  Mode=Multidimensional array
  Matrix Concatenation2 : Concatenate  Mode=Multidimensional array  ConcatenateDimension=2
  R : Selector  NumberOfDimensions=2  InputPortWidth=3  IndexOptions=Index vector (dialog),Index vector (dialog)  Indices=[1,2,3],[1 2 3]  OutputSizes=1
  p : Selector  NumberOfDimensions=2  InputPortWidth=3  IndexOptions=Index vector (dialog),Index vector (dialog)  Indices=[1 2 3],4  OutputSizes=1
  inv(AdH) : Outport  OutDataType=sfix(16)  OutScaling=2^0
  wires:
  R/1 -> Math Function/1
  p/1 -> Cross-Product/2(v)
  H/1 -> R/1, p/1
  0/1 -> Matrix Concatenation2/1
  Matrix Concatenation/1 -> Matrix Concatenation1/1
  Cross-Product/1(out) -> Gain/1
  Matrix Concatenation2/1 -> Matrix Concatenation1/2
  Matrix Concatenation1/1 -> inv(AdH)/1
  Math Function/1 -> Matrix Concatenation/1, Cross-Product/1(m), Matrix Concatenation2/2
  Gain/1 -> Matrix Concatenation/2

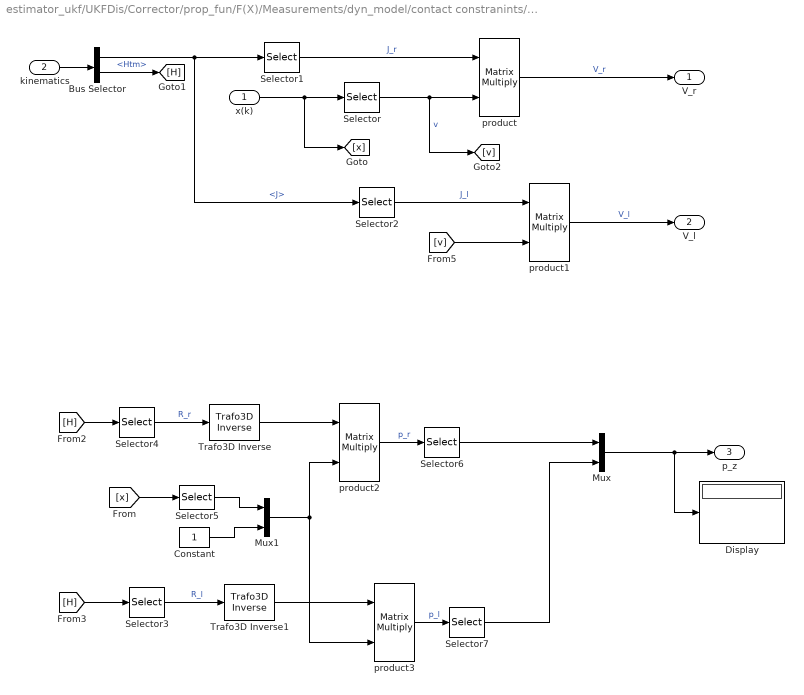
== system estimator_ukf/UKFDis/Corrector/prop_fun/F(X)/Measurements/dyn_model/contact constranints/DoubleSupport ==
  x(k) : Inport  OutDataType=sfix(16)  OutScaling=2^0
  kinematics : Inport  Port=2  OutDataType=sfix(16)  OutScaling=2^0
  Bus Selector : BusSelector  OutputSignals=J,Htm
  Constant : Constant  OutDataType=sfix(16)  OutScaling=2^0
  Display : Display
  Mux : Mux  Inputs=2
  Mux1 : Mux  Inputs=2
  Selector : Selector  InputPortWidth=62  IndexOptions=Index vector (dialog)  Indices=[32:62]  OutputSizes=1
  Selector1 : Selector  NumberOfDimensions=2  InputPortWidth=62  IndexOptions=Index vector (dialog),Select all  Indices=[1:6],1  OutputSizes=1,1
  Selector2 : Selector  NumberOfDimensions=2  InputPortWidth=62  IndexOptions=Index vector (dialog),Select all  Indices=[7:12],1  OutputSizes=1,1
  Selector3 : Selector  NumberOfDimensions=2  InputPortWidth=62  IndexOptions=Index vector (dialog),Select all  Indices=[5:8],[1:3]  OutputSizes=1,1
  Selector4 : Selector  NumberOfDimensions=2  InputPortWidth=62  IndexOptions=Index vector (dialog),Select all  Indices=[1:4],[1:3]  OutputSizes=1,1
  Selector5 : Selector  InputPortWidth=62  IndexOptions=Index vector (dialog)  Indices=[1:3]  OutputSizes=1
  Selector6 : Selector  InputPortWidth=3  IndexOptions=Index vector (dialog)  Indices=[3]  OutputSizes=1
  Selector7 : Selector  InputPortWidth=3  IndexOptions=Index vector (dialog)  Indices=[3]  OutputSizes=1
  Trafo3D Inverse : robotics/Trafo3D Inverse  SystemSampleTime=-1
  Trafo3D Inverse1 : robotics/Trafo3D Inverse  SystemSampleTime=-1
  product{,1..3} (4 alike) : Product  Inputs=**  Multiplication=Matrix(*)  OutDataType=sfix(16)  OutScaling=2^-10
  V_r : Outport  OutDataType=sfix(16)  OutScaling=2^0
  V_l : Outport  Port=2  OutDataType=sfix(16)  OutScaling=2^0
  p_z : Outport  Port=3  OutDataType=sfix(16)  OutScaling=2^0
  wires:
  product1/1 -> V_l/1  "V_l"
  kinematics/1 -> Bus Selector/1
  Selector/1 -> [v], product/2  "v"
  product/1 -> V_r/1  "V_r"
  Bus Selector/1 -> Selector1/1, Selector2/1  "<J>"
  Bus Selector/2 -> [H]  "<Htm>"
  product3/1 -> Selector7/1  "p_l"
  Selector4/1 -> Trafo3D Inverse/1  "R_r"
  [x] -> Selector5/1
  Selector3/1 -> Trafo3D Inverse1/1  "R_l"
  Trafo3D Inverse1/1 -> product3/1
  product2/1 -> Selector6/1  "p_r"
  Selector7/1 -> Mux/2
  Selector6/1 -> Mux/1
  Mux/1 -> p_z/1, Display/1
  x(k)/1 -> Selector/1, [x]
  [H] -> Selector4/1
  [H] -> Selector3/1
  [v] -> product1/2
  Selector1/1 -> product/1  "J_r"
  Selector2/1 -> product1/1  "J_l"
  Selector5/1 -> Mux1/1
  Constant/1 -> Mux1/2
  Mux1/1 -> product2/2, product3/2
  Trafo3D Inverse/1 -> product2/1

== system estimator_ukf/UKFDis/Corrector/prop_fun/F(X)/Measurements/dyn_model/ang rate/Trafo3D Inverse Adjoint/Cross-Product ==
  m : Inport  OutDataType=sfix(16)  OutScaling=2^0
  v : Inport  Port=2  OutDataType=sfix(16)  OutScaling=2^0
  Gain : Gain  Gain=-1  ParameterDataType=sfix(16)  ParameterScaling=2^0  OutDataType=sfix(16)  OutScaling=2^0  SaturateOnIntegerOverflow=on
  Gain1 : Gain  Gain=-1  ParameterDataType=sfix(16)  ParameterScaling=2^0  OutDataType=sfix(16)  OutScaling=2^0  SaturateOnIntegerOverflow=on
  Gain2 : Gain  Gain=-1  ParameterDataType=sfix(16)  ParameterScaling=2^0  OutDataType=sfix(16)  OutScaling=2^0  SaturateOnIntegerOverflow=on
  Matrix Concatenation1 : Concatenate  NumInputs=3  Mode=Multidimensional array
  Matrix Concatenation2 : Concatenate  NumInputs=3  Mode=Multidimensional array
  Matrix Concatenation3 : Concatenate  NumInputs=3  Mode=Multidimensional array
  Matrix Concatenation4 : Concatenate  NumInputs=3  Mode=Multidimensional array  ConcatenateDimension=2
  Product : Product  Multiplication=Matrix(*)  OutDataType=sfix(16)  OutScaling=2^0  SaturateOnIntegerOverflow=on  InputSameDT=on
  Selector : Selector  InputPortWidth=3  IndexOptions=Index vector (dialog)  Indices=[1]  OutputSizes=1
  Selector1 : Selector  InputPortWidth=3  IndexOptions=Index vector (dialog)  Indices=[2]  OutputSizes=1
  Selector2 : Selector  InputPortWidth=3  IndexOptions=Index vector (dialog)  Indices=[3]  OutputSizes=1
  zero : Constant  Value=0  OutDataType=sfix(16)  OutScaling=2^0
  out : Outport  OutDataType=sfix(16)  OutScaling=2^0
  wires:
  zero/1 -> Matrix Concatenation2/1, Matrix Concatenation1/2, Matrix Concatenation3/3
  Selector/1 -> Gain/1, Matrix Concatenation1/3
  Selector1/1 -> Gain1/1, Matrix Concatenation3/1
  Selector2/1 -> Gain2/1, Matrix Concatenation2/2
  Gain1/1 -> Matrix Concatenation2/3
  Gain2/1 -> Matrix Concatenation1/1
  Matrix Concatenation2/1 -> Matrix Concatenation4/1
  Matrix Concatenation1/1 -> Matrix Concatenation4/2
  Matrix Concatenation3/1 -> Matrix Concatenation4/3
  Gain/1 -> Matrix Concatenation3/2
  v/1 -> Selector/1, Selector1/1, Selector2/1
  Product/1 -> out/1
  m/1 -> Product/1
  Matrix Concatenation4/1 -> Product/2

== matlab function UKFDis/Predictor/Embedded MATLAB Function1 ==
  data: M input inherited; X output inherited; Pu input inherited; c input inherited
function X = ut_sigmas(M,Pu,c)

%A = chol(Pu)';

%%{
  A = Pu;
  L  = zeros(size(A));
  def = 1;
  for i=1:size(A,1)
      for j=1:i
          s = A(i,j);
          for k=1:j-1
              s = s - L(i,k)*L(j,k);
          end
          if j < i
              if L(j,j) > eps
                  L(i,j) = s / L(j,j);
              else
                  L(i,j) = 0;
              end
          else
              if (s < -eps)
                  s = 0;
                  def = -1;
              elseif (s < eps)
                  s = 0;
                  def = min(0,def);
              end
              L(j,j) = sqrt(s);
          end
      end
  end
  A = L;
 %%}
  X = [zeros(size(M)) A -A];
  X = sqrt(c)*X + repmat(M,1,size(X,2));

== matlab function UKFDis/Corrector/Embedded MATLAB Function1 ==
  data: M input inherited; X output inherited; Pu input inherited; c input inherited
function X = ut_sigmas(M,Pu,c)

%A = chol(Pu)';

%%{
  A = Pu;
  L  = zeros(size(A));
  def = 1;
  for i=1:size(A,1)
      for j=1:i
          s = A(i,j);
          for k=1:j-1
              s = s - L(i,k)*L(j,k);
          end
          if j < i
              if L(j,j) > eps
                  L(i,j) = s / L(j,j);
              else
                  L(i,j) = 0;
              end
          else
              if (s < -eps)
                  s = 0;
                  def = -1;
              elseif (s < eps)
                  s = 0;
                  def = min(0,def);
              end
              L(j,j) = sqrt(s);
          end
      end
  end
  A = L;
 %%}
  X = [zeros(size(M)) A -A];
  X = sqrt(c)*X + repmat(M,1,size(X,2));
